simulink library "DYN_TRA"  (Simulink 9.0)
settings: Solver=ode45  StartTime=0.0  StopTime=10.0  RelTol=1e-3  EnableMultiTasking=on
libraries: LIB_ROT x2, LIB_DYN x1, LIB_ORB x1
settings Model: Creator=alger  LastModifiedBy=Mike

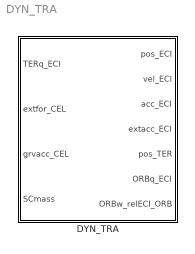
== system DYN_TRA ==
  "DYN_TRA " : Subsystem

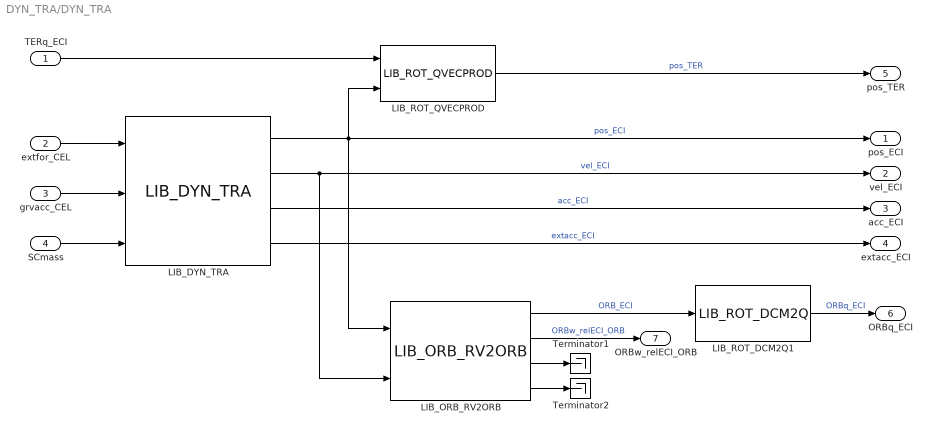
== system DYN_TRA/DYN_TRA  ==
  TERq_ECI : Inport  PortDimensions=4
  extfor_CEL : Inport  Port=2  PortDimensions=3
  grvacc_CEL : Inport  Port=3  PortDimensions=3
  SCmass : Inport  Port=4  PortDimensions=1
  LIB_DYN_TRA : LIB_DYN/LIB_DYN_TRA  pos_CEL_ini=DYN_TRA_par.pos_ECI_ini  vel_CEL_ini=DYN_TRA_par.vel_ECI_ini
  LIB_ORB_RV2ORB : LIB_ORB/LIB_ORB_RV2ORB  tol=CONSTANTS_par.zero_tol
  LIB_ROT_DCM2Q1 : LIB_ROT/LIB_ROT_DCM2Q
  LIB_ROT_QVECPROD : LIB_ROT/LIB_ROT_QVECPROD
  Terminator1 : Terminator
  Terminator2 : Terminator
  pos_ECI : Outport  PortDimensions=3
  vel_ECI : Outport  Port=2  PortDimensions=3
  acc_ECI : Outport  Port=3  PortDimensions=3
  extacc_ECI : Outport  Port=4  PortDimensions=3
  pos_TER : Outport  Port=5  PortDimensions=3
  ORBq_ECI : Outport  Port=6  PortDimensions=4
  ORBw_relECI_ORB : Outport  Port=7  PortDimensions=3
  wires:
  extfor_CEL/1 -> LIB_DYN_TRA/1
  LIB_DYN_TRA/3 -> acc_ECI/1  "acc_ECI"
  LIB_DYN_TRA/4 -> extacc_ECI/1  "extacc_ECI"
  SCmass/1 -> LIB_DYN_TRA/3
  TERq_ECI/1 -> LIB_ROT_QVECPROD/1
  grvacc_CEL/1 -> LIB_DYN_TRA/2
  LIB_ROT_QVECPROD/1 -> pos_TER/1  "pos_TER"
  LIB_DYN_TRA/2 -> LIB_ORB_RV2ORB/2, vel_ECI/1  "vel_ECI"
  LIB_DYN_TRA/1 -> LIB_ROT_QVECPROD/2, LIB_ORB_RV2ORB/1, pos_ECI/1  "pos_ECI"
  LIB_ORB_RV2ORB/3 -> Terminator1/1
  LIB_ORB_RV2ORB/1 -> LIB_ROT_DCM2Q1/1  "ORB_ECI"
  LIB_ORB_RV2ORB/4 -> Terminator2/1
  LIB_ROT_DCM2Q1/1 -> ORBq_ECI/1  "ORBq_ECI"
  LIB_ORB_RV2ORB/2 -> ORBw_relECI_ORB/1  "ORBw_relECI_ORB"
